simulink model "gm_test1"  (R2023b)
settings: Solver=VariableStepAuto  StartTime=0.0  StopTime=100000  RelTol=1e-3
undefined symbols (not defined in the file or in its folder): bhi, cnt1_max
libraries: hdlsllib x2, dsphdlfiltering2 x1
settings Model: Creator=31651  LastModifiedBy=31651
settings OptimizationCC: BlockReduction=off  ConditionallyExecuteInputs=off  DefaultParameterBehavior=Inlined
settings DebuggingCC: AlgebraicLoopMsg=error  InheritedTsInSrcMsg=none
settings HardwareCC: ProdBitPerPointer=32  ProdBitPerSizeT=32  ProdBitPerPtrDiffT=32  ProdLargestAtomicFloat=None  ProdIntDivRoundTo=Undefined  ProdEndianess=Unspecified  ProdWordSize=32  ProdHWDeviceType=ASIC/FPGA->ASIC/FPGA  TargetBitPerPointer=64  TargetBitPerSizeT=64  TargetBitPerPtrDiffT=64  TargetLongLongMode=on  TargetIntDivRoundTo=Zero  TargetEndianess=LittleEndian  TargetWordSize=64  TargetHWDeviceType=Custom Processor->MATLAB Host Computer  ProdEqTarget=off

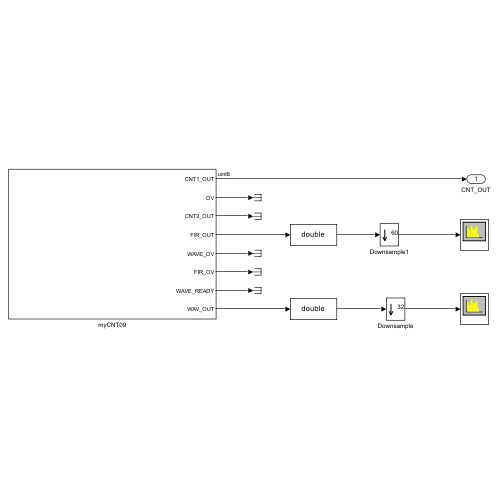
[thumbnail: Simulink's stored preview of the top-level diagram]
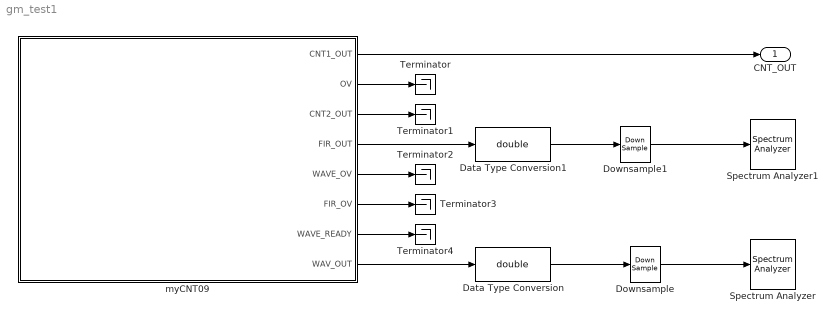
== system gm_test1 ==
  Data Type Conversion : DataTypeConversion  OutDataTypeStr=double  SaturateOnIntegerOverflow=off  RndMeth=Floor  LockScale=on
  Data Type Conversion1 : DataTypeConversion  OutDataTypeStr=double  SaturateOnIntegerOverflow=off  RndMeth=Floor  LockScale=on
  Downsample : DownSample  N=32  RateOptions=Allow multirate processing
  Downsample1 : DownSample  N=60  RateOptions=Allow multirate processing
  Spectrum Analyzer : SpectrumAnalyzer  WindowPosition=[368.000000,182.000000,800.000000,500.000000,]  Visible=on  ScopeFrameLocation=window  YLimits=[-157.22656225,-41.1761275]
  Spectrum Analyzer1 : SpectrumAnalyzer  WindowPosition=[235.000000,112.000000,800.000000,500.000000,]  Visible=on  ScopeFrameLocation=window  YLimits=[-3603.44492261,-2802.67938425]
  Terminator{,1..4} (5 alike) : Terminator
  myCNT09 : Subsystem
  CNT_OUT : Outport  VectorParamsAs1DForOutWhenUnconnected=off
  wires:
  Downsample1/1 -> Spectrum Analyzer1/1
  myCNT09/6(FIR_OV) -> Terminator3/1
  myCNT09/7(WAVE_READY) -> Terminator4/1
  myCNT09/4(FIR_OUT) -> Data Type Conversion1/1
  Data Type Conversion1/1 -> Downsample1/1
  myCNT09/8(WAV_OUT) -> Data Type Conversion/1
  Data Type Conversion/1 -> Downsample/1
  Downsample/1 -> Spectrum Analyzer/1
  myCNT09/5(WAVE_OV) -> Terminator2/1
  myCNT09/2(OV) -> Terminator/1
  myCNT09/3(CNT2_OUT) -> Terminator1/1
  myCNT09/1(CNT1_OUT) -> CNT_OUT/1

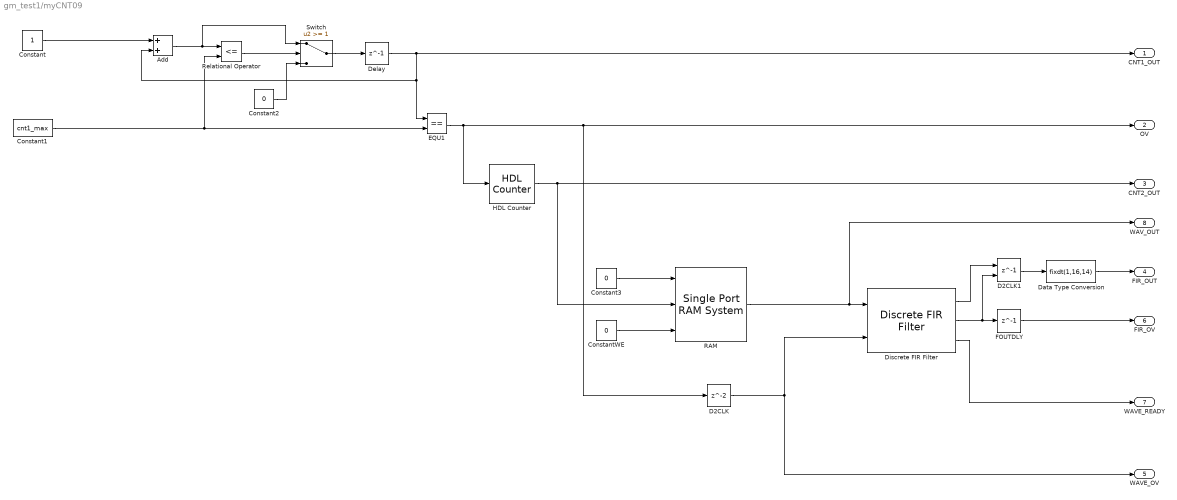
== system gm_test1/myCNT09 ==
  Add : Sum  OutDataTypeStr=uint8
  Constant : Constant  OutDataTypeStr=uint8  SampleTime=1
  Constant1 : Constant  Value=cnt1_max  OutDataTypeStr=uint8  SampleTime=1
  Constant2 : Constant  Value=0  OutDataTypeStr=uint8  SampleTime=1
  Constant3 : Constant  Value=0  OutDataTypeStr=fixdt(1,16,15)  SampleTime=1
  ConstantWE : Constant  Value=0  OutDataTypeStr=boolean  SampleTime=1
  D2CLK : Delay  InitialCondition=0
  D2CLK1 : Delay  DelayLength=1  InitialCondition=0  ShowEnablePort=on
      settings: InputPortMap=u0,e6
  Data Type Conversion : DataTypeConversion  OutDataTypeStr=fixdt(1,16,14)  SaturateOnIntegerOverflow=off  RndMeth=Floor
  Delay : Delay  DelayLength=1  InitialCondition=0
  Discrete FIR Filter : dsphdlfiltering2/Discrete FIR Filter  NumeratorSource=Property  Numerator=bhi  NumeratorPrototype=[]  FilterStructure=Partly serial systolic  SerializationOption=Maximum number of multipliers  NumCycles=2  NumberOfMultipliers=3  SimulateUsing=Code generation  roundingMode=Floor  overflowMode=off  CoefficientsDataTypeStr=Inherit: Same word length as input  OutputDataTypeStr=Inherit: Same word length as input  ResetInputPort=off  HDLGlobalReset=off  CoeffMultiplier=Multiplier  UseMultForPow2Coeff=on
  EQU1 : RelationalOperator  Operator===  InputSameDT=off
  FOUTDLY : Delay  DelayLength=1  InitialCondition=0
  HDL Counter : hdlsllib/Sources/HDL Counter  CountType=Count limited  CountInit=0  CountStep=1  CountMax=cnt2_max  CountFromType=Initial value  CountFrom=0  CountResetPort=off  CountLoadPort=off  CountEnbPort=on  CountDirPort=off  CountHitOutputPort=off  CountDataType=Unsigned  CountWordLen=8  CountFracLen=0  CountSampTime=1
  RAM : hdlsllib/HDL RAMs/Single Port RAM System  RAMType=Single port  AsyncRead=off  WriteOutputValue=New data  RAMInitialValue=vec_ram_fix  allowBusInputs=off  WritesHaveOutput=on  NumReads=0  NumWrites=1  SimulateUsing=Code generation
  Relational Operator : RelationalOperator  Operator=<=  OutDataTypeStr=boolean  InputSameDT=off
  Switch : Switch  Threshold=1  OutDataTypeStr=uint8  SaturateOnIntegerOverflow=off  InputSameDT=off
  CNT1_OUT : Outport  OutDataTypeStr=uint8  VectorParamsAs1DForOutWhenUnconnected=off
  OV : Outport  Port=2  VectorParamsAs1DForOutWhenUnconnected=off
  CNT2_OUT : Outport  Port=3
  FIR_OUT : Outport  Port=4  VectorParamsAs1DForOutWhenUnconnected=off
  WAVE_OV : Outport  Port=5  VectorParamsAs1DForOutWhenUnconnected=off
  FIR_OV : Outport  Port=6  VectorParamsAs1DForOutWhenUnconnected=off
  WAVE_READY : Outport  Port=7  VectorParamsAs1DForOutWhenUnconnected=off
  WAV_OUT : Outport  Port=8
  wires:
  Data Type Conversion/1 -> FIR_OUT/1
  RAM/1 -> Discrete FIR Filter/1, WAV_OUT/1
  FOUTDLY/1 -> FIR_OV/1
  D2CLK1/1 -> Data Type Conversion/1
  Discrete FIR Filter/3 -> WAVE_READY/1
  Discrete FIR Filter/2 -> D2CLK1/2, FOUTDLY/1
  D2CLK/1 -> WAVE_OV/1, Discrete FIR Filter/2
  Discrete FIR Filter/1 -> D2CLK1/1
  Constant3/1 -> RAM/1
  ConstantWE/1 -> RAM/3
  HDL Counter/1 -> CNT2_OUT/1, RAM/2
  EQU1/1 -> OV/1, D2CLK/1, HDL Counter/1
  Constant2/1 -> Switch/3
  Constant1/1 -> EQU1/2, Relational Operator/2
  Constant/1 -> Add/1
  Delay/1 -> CNT1_OUT/1, Add/2, EQU1/1
  Add/1 -> Relational Operator/1, Switch/1
  Relational Operator/1 -> Switch/2
  Switch/1 -> Delay/1
